simulink model "modulator_demodulator_postfig_7"  (R2021b)
settings: Solver=VariableStepAuto  StartTime=0.0  StopTime=1.5  RelTol=1e-3
undefined symbols (not defined in the file): magnitude
libraries: dsparch4 x1
settings Model: Creator=Joshua  LastModifiedBy=Joshua

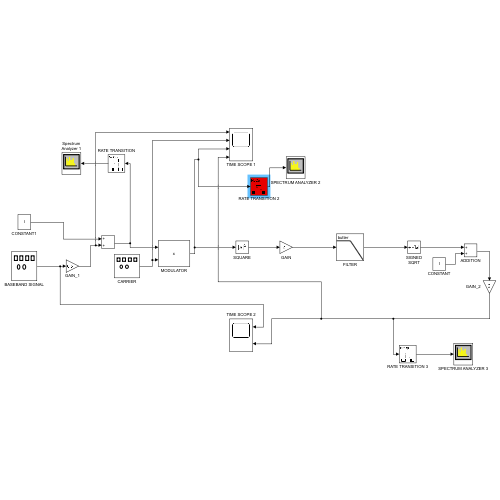
[thumbnail: Simulink's stored preview of the top-level diagram]
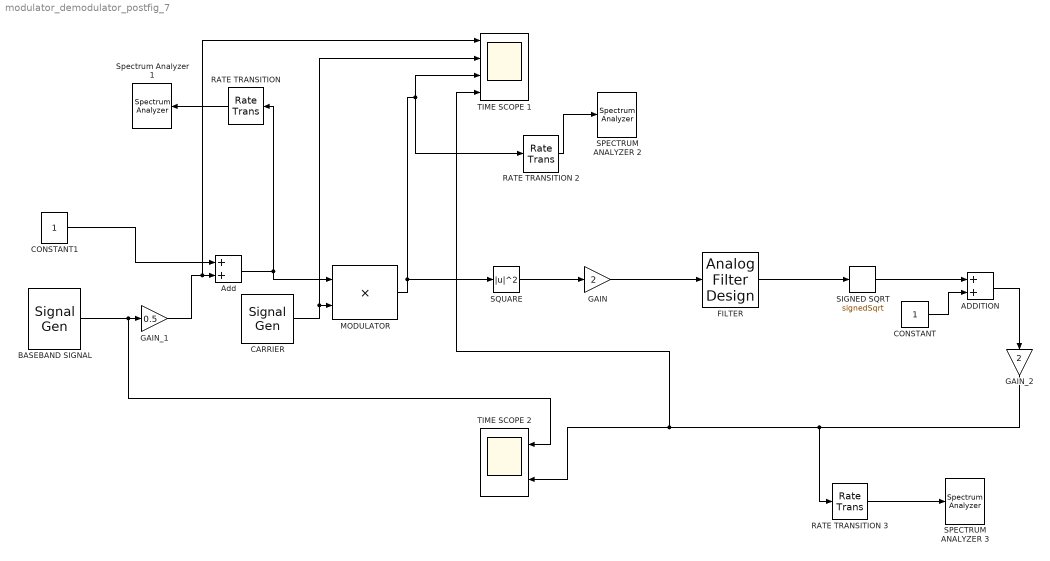
== system modulator_demodulator_postfig_7 ==
  ADDITION : Sum
  Add : Sum
  BASEBAND SIGNAL : SignalGenerator  Frequency=1000
  CARRIER : SignalGenerator  Frequency=20000
  CONSTANT : Constant
  CONSTANT1 : Constant
  FILTER : dsparch4/Analog Filter Design  method=Butterworth  filttype=Lowpass  N=8  Wlo=2*pi*11000  Whi=80  Rp=2  Rs=40
  GAIN : Gain  Gain=2
  GAIN_1 : Gain  Gain=0.5
  GAIN_2 : Gain  Gain=2
  MODULATOR : Product
  RATE TRANSITION : RateTransition  OutPortSampleTimeOpt=Inherit
  RATE TRANSITION 2 : RateTransition
  RATE TRANSITION 3 : RateTransition
  SIGNED SQRT : Sqrt  Operator=signedSqrt  SaturateOnIntegerOverflow=on
  SPECTRUM ANALYZER 2 : SpectrumAnalyzer
  SPECTRUM ANALYZER 3 : SpectrumAnalyzer
  SQUARE : Math  Operator=magnitude^2  SaturateOnIntegerOverflow=on
  Spectrum Analyzer 1 : SpectrumAnalyzer
  TIME SCOPE 1 : Scope  NumInputPorts=4
  TIME SCOPE 2 : Scope  NumInputPorts=2
  wires:
  CARRIER/1 -> TIME SCOPE 1/2, MODULATOR/2
  MODULATOR/1 -> SQUARE/1, RATE TRANSITION 2/1, TIME SCOPE 1/3
  SQUARE/1 -> GAIN/1
  GAIN/1 -> FILTER/1
  FILTER/1 -> SIGNED SQRT/1
  CONSTANT/1 -> ADDITION/2
  SIGNED SQRT/1 -> ADDITION/1
  BASEBAND SIGNAL/1 -> TIME SCOPE 2/1, GAIN_1/1
  GAIN_1/1 -> TIME SCOPE 1/1, Add/2
  Add/1 -> RATE TRANSITION/1, MODULATOR/1
  CONSTANT1/1 -> Add/1
  RATE TRANSITION/1 -> Spectrum Analyzer 1/1
  ADDITION/1 -> GAIN_2/1
  GAIN_2/1 -> RATE TRANSITION 3/1, TIME SCOPE 1/4, TIME SCOPE 2/2
  RATE TRANSITION 3/1 -> SPECTRUM ANALYZER 3/1
  RATE TRANSITION 2/1 -> SPECTRUM ANALYZER 2/1
